simulink model "controller"  (R2021b)
settings: Solver=FixedStepDiscrete  StartTime=0.0  StopTime=10.0  FixedStep=1/1000  RelTol=1e-3  EnableMultiTasking=on
libraries: simulink x4
settings Model: ExtModeTrigDuration=2  Creator=DAUIN-Win10  LastModifiedBy=maria
settings OptimizationCC: EnhancedBackFolding=on  PassReuseOutputArgsAs=Individual arguments  ZeroExternalMemoryAtStartup=off  ZeroInternalMemoryAtStartup=off  MaxStackSize=64  OptimizeBlockOrder=speed  DifferentSizesBufferReuse=on  OptimizationCustomize=off  EfficientTunableParamExpr=on
settings DebuggingCC: ParameterTunabilityLossMsg=error
settings HardwareCC: ProdBitPerInt=16  ProdBitPerPointer=16  ProdBitPerSizeT=16  ProdBitPerPtrDiffT=16  ProdLargestAtomicFloat=None  ProdWordSize=8  ProdHWDeviceType=Atmel->AVR
settings SFSimCC: MATLABDynamicMemAlloc=off
settings RTWCC: Description=Embedded Coder  SystemTargetFile=ert.tlc  HardwareBoard=Arduino Uno  TemplateMakefile=ert_default_tmf  Toolchain=Arduino AVR  BuildConfiguration=Faster Runs
settings CodeAppCC: ForceParamTrailComments=on  IgnoreCustomStorageClasses=off  OperatorAnnotations=on  SimulinkDataObjDesc=on  SFDataObjDesc=on  InsertBlockDesc=on
settings ERTTargetCC: SupportContinuousTime=on  SupportVariableSizeSignals=on  ExtModeTransport=3  ExtModeStaticAlloc=on  ExtModeStaticAllocSize=250  ExtModeMexFile=ext_xcp  ExtModeIntrfLevel=Level2 - Open

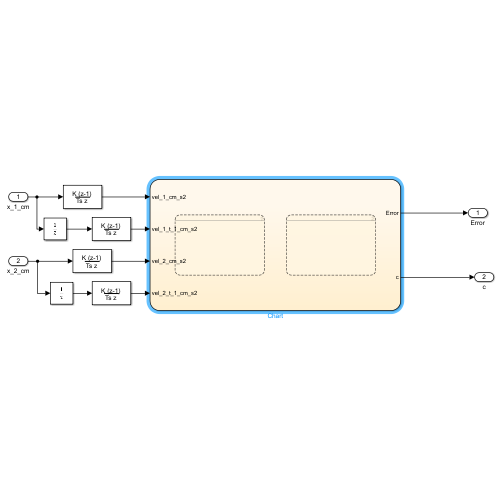
[thumbnail: Simulink's stored preview of the top-level diagram]
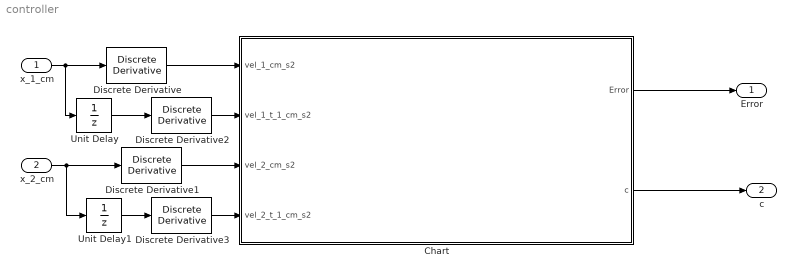
== system controller ==
  x_1_cm : Inport
  x_2_cm : Inport  Port=2
  Chart : Stateflow chart  TreatAsAtomicUnit=on
  Discrete Derivative{,1..3} (4 alike) : simulink/Discrete/Discrete Derivative  gainval=1.0  ICPrevScaledInput=0.0  OutMin=[]  OutMax=[]  OutDataType=fixdt(1, 16)  OutScaling=2^-10  DoSatur=off
  Unit Delay : UnitDelay  SampleTime=-1  HasFrameUpgradeWarning=on
  Unit Delay1 : UnitDelay  SampleTime=-1  HasFrameUpgradeWarning=on
  Error : Outport
  c : Outport  Port=2  OutDataTypeStr=boolean
  wires:
  Unit Delay1/1 -> Discrete Derivative3/1
  x_1_cm/1 -> Unit Delay/1, Discrete Derivative/1
  Discrete Derivative2/1 -> Chart/2(vel_1_t_1_cm_s2)
  Discrete Derivative1/1 -> Chart/3(vel_2_cm_s2)
  Unit Delay/1 -> Discrete Derivative2/1
  Discrete Derivative/1 -> Chart/1(vel_1_cm_s2)
  Discrete Derivative3/1 -> Chart/4(vel_2_t_1_cm_s2)
  x_2_cm/1 -> Unit Delay1/1, Discrete Derivative1/1
  Chart/1(Error) -> Error/1
  Chart/2(c) -> c/1

== stateflow chart controller/Chart ==
  state Skyhook_control_system [parallel]
    settings: executionOrder=1
    state Condition_cl
      entry:
      c = 0;
    state Condition_ch
      entry:
      c = 1;
    (default) -> Condition_ch
    Condition_cl -> Condition_ch : [((vel_1_cm_s2-vel_2_cm_s2)*vel_1_cm_s2)>=0 && Error != 1]
    Condition_ch -> Condition_cl : [((vel_1_cm_s2-vel_2_cm_s2)*vel_1_cm_s2)<0  && Error != 1]
  state Error_Checker [parallel]
    settings: executionOrder=2
    state Vel_1 [parallel]
      settings: executionOrder=1
      state Sensor_ok
        entry:
        Error = 0;
      state Sensor_down
        entry:
        Error = 1;
        c = 1;
      (default) -> Error_Checker.Vel_1.Sensor_ok
      Error_Checker.Vel_1.Sensor_ok -> Error_Checker.Vel_1.Sensor_down : [duration(abs(vel_1_cm_s2-vel_1_t_1_cm_s2)<=2^(-53))>=0.020]
    state Vel_2 [parallel]
      settings: executionOrder=2
      state Sensor_ok
        entry:
        Error = 0;
      state Sensor_down
        entry:
        Error = 1;
        c = 1;
      (default) -> Error_Checker.Vel_2.Sensor_ok
      Error_Checker.Vel_2.Sensor_ok -> Error_Checker.Vel_2.Sensor_down : [duration(abs(vel_2_cm_s2-vel_2_t_1_cm_s2)<=2^(-53))>=0.020]
  data: Error output double; vel_1_cm_s2 input; c output boolean; vel_1_t_1_cm_s2 input; vel_2_cm_s2 input double; vel_2_t_1_cm_s2 input double
